simulink model "E12_implementation"  (R2017a)
settings: Solver=VariableStepAuto  StartTime=0.0  StopTime=100  RelTol=1e-3
InitFcn:
  | clear
  | E_param
undefined symbols (not defined in the file or in its folder): E_animation
settings Model: Creator=Mat Haskell  LastModifiedBy=Mat Haskell

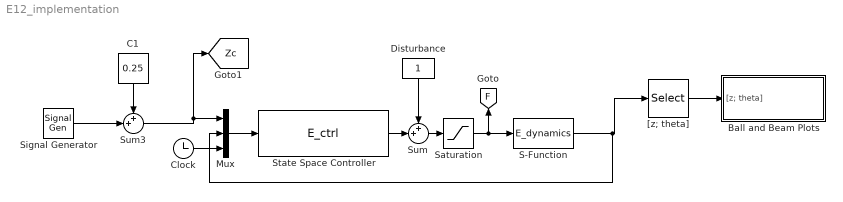
== system E12_implementation ==
  Ball and Beam Plots : Subsystem
  C1 : Constant  Value=0.25
  Clock : Clock
  Disturbance : Constant
  Mux : Mux  Inputs=3
  S-Function : S-Function  FunctionName=E_dynamics  Parameters=P  SFunctionDeploymentMode=off  EnableBusSupport=off
  Saturation : Saturate  UpperLimit=15  LowerLimit=-15
  Signal Generator : SignalGenerator  WaveForm=square  Amplitude=.125  Frequency=.02
  State Space Controller : MATLABFcn  InitFcn=E_param  MATLABFcn=E_ctrl
  Sum : Sum  Inputs=++|
  Sum3 : Sum  Inputs=++|
  "[z; theta]" : Selector  InputPortWidth=4  IndexOptions=Index vector (dialog)  Indices=[1 2]  OutputSizes=1
  tag scope: F=global, Zc=global
  wires:
  Sum3/1 -> [Zc], Mux/1
  Saturation/1 -> S-Function/1, [F]
  C1/1 -> Sum3/1
  Signal Generator/1 -> Sum3/2
  Mux/1 -> State Space Controller/1
  "[z; theta]"/1 -> Ball and Beam Plots/1("[z; theta]")
  S-Function/1 -> Mux/2, "[z; theta]"/1
  State Space Controller/1 -> Sum/2
  Sum/1 -> Saturation/1
  Disturbance/1 -> Sum/1
  Clock/1 -> Mux/3

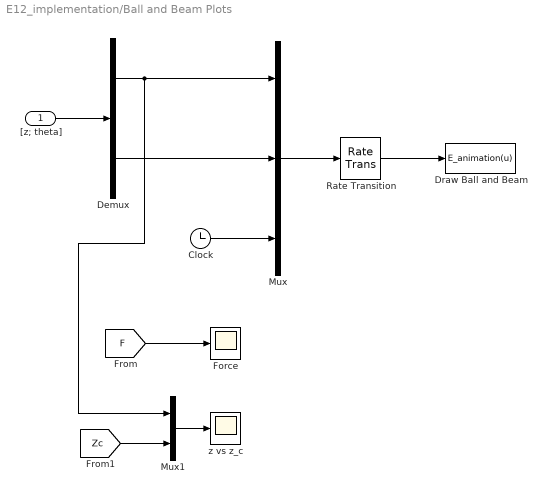
== system E12_implementation/Ball and Beam Plots ==
  "[z; theta]" : Inport
  Clock : Clock
  Demux : Demux  Outputs=2
  Draw Ball and Beam : MATLABFcn  MATLABFcn=E_animation(u)  OutputDimensions=0
  Force : Scope
  Mux : Mux  Inputs=3
  Mux1 : Mux  Inputs=2
  Rate Transition : RateTransition  OutPortSampleTime=P.t_plot
  z vs z_c : Scope
  wires:
  "[z; theta]"/1 -> Demux/1
  Rate Transition/1 -> Draw Ball and Beam/1
  Mux/1 -> Rate Transition/1
  Clock/1 -> Mux/3
  Demux/1 -> Mux1/1, Mux/1
  Demux/2 -> Mux/2
  [F] -> Force/1
  Mux1/1 -> z vs z_c/1
  [Zc] -> Mux1/2
